simulink model "lqr_pos_control"  (R2021a)
settings: Solver=FixedStepAuto  StartTime=0.0  StopTime=inf  FixedStep=.01  RelTol=1e-3
model workspace (MAT data in the model file):
  SL_ROS_VariableLengthArrays_MaxSizes.CommonInfo.ArrayTruncateAction = 'EmitWarning'
  SL_ROS_VariableLengthArrays_MaxSizes.MsgTypeMap = containers.Map
  SL_ROS_VariableLengthArrays_MaxSizes.MsgTypeMap.serialization.keys = {'mav_msgs/Actuators'}
  SL_ROS_VariableLengthArrays_MaxSizes.MsgTypeMap.serialization.values{1}(1).PropertyName = 'Angles'
  SL_ROS_VariableLengthArrays_MaxSizes.MsgTypeMap.serialization.values{1}(1).DataType = 'double'
  SL_ROS_VariableLengthArrays_MaxSizes.MsgTypeMap.serialization.values{1}(1).MaxLength = 128
  SL_ROS_VariableLengthArrays_MaxSizes.MsgTypeMap.serialization.values{1}(2).PropertyName = 'AngularVelocities'
  SL_ROS_VariableLengthArrays_MaxSizes.MsgTypeMap.serialization.values{1}(2).DataType = 'double'
  SL_ROS_VariableLengthArrays_MaxSizes.MsgTypeMap.serialization.values{1}(2).MaxLength = 4
  SL_ROS_VariableLengthArrays_MaxSizes.MsgTypeMap.serialization.values{1}(3).PropertyName = 'Normalized'
  SL_ROS_VariableLengthArrays_MaxSizes.MsgTypeMap.serialization.values{1}(3).DataType = 'double'
  SL_ROS_VariableLengthArrays_MaxSizes.MsgTypeMap.serialization.values{1}(3).MaxLength = 128
  SL_ROS_VariableLengthArrays_MaxSizes.MsgTypeMap.serialization.uniformity = 0
  SL_ROS_VariableLengthArrays_MaxSizes.MsgTypeMap.serialization.keyType = 'char'
  SL_ROS_VariableLengthArrays_MaxSizes.MsgTypeMap.serialization.valueType = 'any'
values from neighbouring files (symbols this model uses):
  airframe = struct()    [discreteModel_initializer.m]
  Fs = 100    [discreteModel_initializer.m]
  g = 9.81    [discreteModel_initializer.m]
  kLQR = dlqr(lqrDiscrete.A,lqrDiscrete.B,Q,R)    [discreteModel_initializer.m]
  Ts = 1/Fs    (= 0.01)    [discreteModel_initializer.m]
  wiHover = sqrt(((airframe.mass)*9.81)/(4*airframe.Propeller.Ct))    [discreteModel_initializer.m]
undefined symbols (not defined in the file or in its folder): DiscIntNeverNeededParam, Discrete, Gyro_pitch, Gyro_roll, P00, P01, P11, Qkalman, Rkalman, RPM_to_DC, rpmKnown_throttleUnknown, sigbuilder_block, tf1, Time
libraries: robotlib x11, arduinolib x6, sharedtransform x3, simulink x3, ctrlSharedLib x1
(part 1 of 2)
settings Model: SILPILModeSetting=veronly  EnablePacing=on  ExtModeTrigDuration=2  Creator=aaron  LastModifiedBy=aaron
settings OptimizationCC: EnhancedBackFolding=on  PassReuseOutputArgsAs=Individual arguments  ZeroExternalMemoryAtStartup=off  ZeroInternalMemoryAtStartup=off  MaxStackSize=64  OptimizeBlockOrder=speed  DifferentSizesBufferReuse=on  OptimizationCustomize=off  EfficientTunableParamExpr=on
settings DebuggingCC: ParameterTunabilityLossMsg=error  UnderSpecifiedDimensionMsg=warning
settings HardwareCC: ProdBitPerPointer=32  ProdBitPerSizeT=32  ProdBitPerPtrDiffT=32  ProdLargestAtomicFloat=None  ProdIntDivRoundTo=Undefined  ProdEndianess=Unspecified  ProdWordSize=32  ProdHWDeviceType=Generic->Unspecified (assume 32-bit Generic)
settings SFSimCC: MATLABDynamicMemAlloc=off
settings RTWCC: SystemTargetFile=ert.tlc  HardwareBoard=Robot Operating System (ROS)  TLCOptions="-aInlineSetEventsForThisBaseRateFcn=TLC_FALSE -aSuppressMultiTaskScheduler=TLC_FALSE    -aRateBasedStepFcn=0"  TemplateMakefile=ert_default_tmf  Toolchain=Catkin  BuildConfiguration=Faster Runs  TargetLang=C++
settings CodeAppCC: ForceParamTrailComments=on  IgnoreCustomStorageClasses=off  OperatorAnnotations=on  SimulinkDataObjDesc=on  SFDataObjDesc=on  InsertBlockDesc=on
settings ERTTargetCC: SupportContinuousTime=on  ExtModeStaticAllocSize=24576

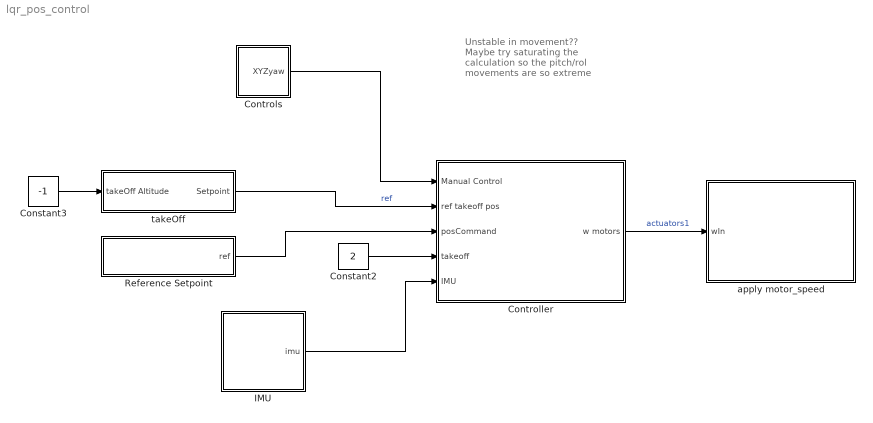
== system lqr_pos_control ==
  note: Unstable in movement??
      | Maybe try saturating the calculation so the pitch/rol movements are so extreme
  Constant2 : Constant  Value=2
  Constant3 : Constant  Value=-1
  Controller : Subsystem
  Controls : Subsystem
  IMU : Subsystem
  Reference Setpoint : Subsystem
  apply motor_speed : Subsystem
  takeOff : Subsystem
  wires:
  Controls/1(XYZyaw) -> Controller/1(Manual Control)
  takeOff/1(Setpoint) -> Controller/2(ref takeoff pos)  "ref"
  Constant3/1 -> takeOff/1(takeOff Altitude)
  Controller/1(w motors) -> apply motor_speed/1(wIn)  "actuators1"
  Constant2/1 -> Controller/4(takeoff)
  IMU/1(imu) -> Controller/5(IMU)
  Reference Setpoint/1(ref) -> Controller/3(posCommand)

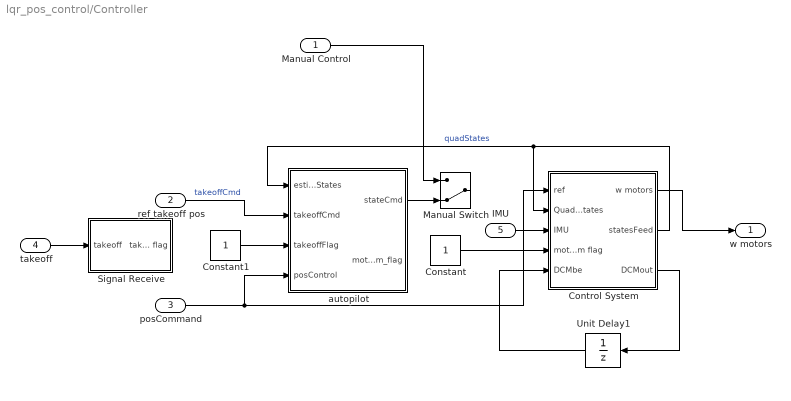
== system lqr_pos_control/Controller ==
  Manual Control : Inport
  ref takeoff pos : Inport  Port=2
  posCommand : Inport  Port=3
  takeoff : Inport  Port=4
  IMU : Inport  Port=5
  Constant : Constant
  Constant1 : Constant
  Control System : Subsystem
  Manual Switch : ManualSwitch  CurrentSetting=0
  Signal Receive : Subsystem
  Unit Delay1 : UnitDelay  InitialCondition=eye(3)  SampleTime=-1  HasFrameUpgradeWarning=on
  autopilot : Stateflow chart  TreatAsAtomicUnit=on
  w motors : Outport
  wires:
  autopilot/1(stateCmd) -> Manual Switch/2
  Manual Control/1 -> Manual Switch/1
  Control System/3(DCMout) -> Unit Delay1/1
  Control System/1(w motors) -> w motors/1
  IMU/1 -> Control System/3(IMU)
  posCommand/1 -> Control System/1(ref), autopilot/4(posControl)
  ref takeoff pos/1 -> autopilot/2(takeoffCmd)  "takeoffCmd"
  Control System/2(statesFeed) -> Control System/2(Quad States), autopilot/1(estimatedStates)  "quadStates"
  Unit Delay1/1 -> Control System/5(DCMbe)
  takeoff/1 -> Signal Receive/1(takeoff)
  Constant/1 -> Control System/4(motor arm flag)
  Constant1/1 -> autopilot/3(takeoffFlag)

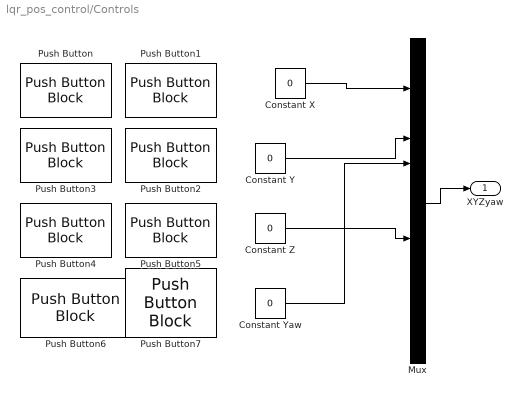
== system lqr_pos_control/Controls ==
  Constant X : Constant  Value=0
  Constant Y : Constant  Value=0
  Constant Yaw : Constant  Value=0
  Constant Z : Constant  Value=0
  Mux : Mux  Inputs=12
  Push Button : PushButtonBlock  LabelPosition=Top  ButtonText=Forward
  Push Button1 : PushButtonBlock  LabelPosition=Top  ButtonText=Backward  OnValue=-1
  Push Button2 : PushButtonBlock  LabelPosition=Top  ButtonText=Right
  Push Button3 : PushButtonBlock  LabelPosition=Top  ButtonText=Left  OnValue=-1
  Push Button4 : PushButtonBlock  LabelPosition=Top  ButtonText=Down  OnValue=-3
  Push Button5 : PushButtonBlock  LabelPosition=Top  ButtonText=Up  OnValue=3
  Push Button6 : PushButtonBlock  LabelPosition=Top  ButtonText=Counterclockwise  OnValue=-1
  Push Button7 : PushButtonBlock  LabelPosition=Top  ButtonText=Clockwise
  XYZyaw : Outport
  wires:
  Mux/1 -> XYZyaw/1
  Constant Yaw/1 -> Mux/5
  Constant X/1 -> Mux/2
  Constant Y/1 -> Mux/4
  Constant Z/1 -> Mux/8

== system lqr_pos_control/IMU ==
  Gain : Gain  Gain=-1
  Mux : Mux  Inputs=6
  Subscribe : robotlib/Subscribe  topicSource=Select from ROS network  topic=/hummingbird/imu  messageType=sensor_msgs/Imu  SampleTime=-1  legacyBusStruct=off  messageQueueLength=1
  Subsystem : Subsystem
  imu : Outport
  wires:
  Subsystem/5(<Y>1) -> Mux/5
  Subsystem/2(<Y>) -> Mux/2
  Subsystem/4(<X>1) -> Mux/4
  Subsystem/6(<Z>1) -> Mux/6
  Subscribe/1 -> Subsystem/Enable
  Subsystem/3(<Z>) -> Gain/1
  Subsystem/1(<X>) -> Mux/1
  Gain/1 -> Mux/3
  Subscribe/2 -> Subsystem/1(In1)
  Mux/1 -> imu/1  "imu"

== system lqr_pos_control/Reference Setpoint ==
  Subscribe4 : robotlib/Subscribe  topicSource=Select from ROS network  topic=/hummingbird/command/pose  messageType=geometry_msgs/PoseStamped  SampleTime=-1  legacyBusStruct=off  messageQueueLength=1
  Subsystem4 : Subsystem
  posControl : Subsystem
  ref : Outport
  wires:
  Subsystem4/3(cmdZ) -> posControl/3(cmdZ)
  Subsystem4/1(cmdX) -> posControl/1(cmdX)
  Subsystem4/4(quatOut) -> posControl/4(cmdAngle)
  Subscribe4/2 -> Subsystem4/1(In1)
  Subscribe4/1 -> Subsystem4/Enable
  Subsystem4/2(cmdY) -> posControl/2(cmdY)
  posControl/1(Setpoint) -> ref/1  "ref"

== system lqr_pos_control/apply motor_speed ==
  wIn : Inport
  MATLAB Function : MATLAB Function  TreatAsAtomicUnit=on
  Publish1 : robotlib/Publish  topicSource=Select from ROS network  topic=/hummingbird/command/motor_speed  messageType=mav_msgs/Actuators  legacyBusStruct=off  messageQueueLength=1
  Subscribe : robotlib/Subscribe  topicSource=Select from ROS network  topic=/hummingbird/motor_speed  messageType=mav_msgs/Actuators  SampleTime=-1  legacyBusStruct=off  messageQueueLength=1
  Subsystem : Subsystem
  wires:
  Subscribe/2 -> Subsystem/1(In1)
  Subscribe/1 -> Subsystem/Enable
  wIn/1 -> MATLAB Function/2(angVel)
  Subsystem/1(<AngularVelocities>) -> MATLAB Function/1(Bus)
  MATLAB Function/1(msg) -> Publish1/1

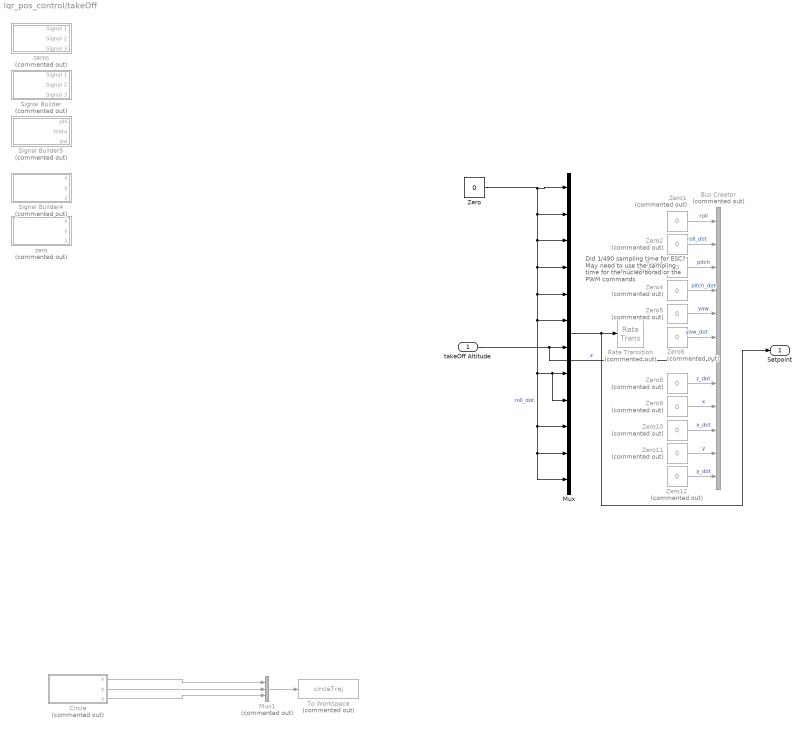
== system lqr_pos_control/takeOff ==
  note: Did 1/490 sampling time for ESC? May need to use the sampling time
      | for the nucleo borad or the PWM commands
  takeOff Altitude : Inport
  Bus Creator : BusCreator  Commented=on  Inputs=12
  Circle : Subsystem  Tag=STV Subsys  Commented=on  LoadFcn=sigbuilder_block('load');  StartFcn=sigbuilder_block('start');  StopFcn=sigbuilder_block('stop');  ClipboardFcn=sigbuilder_block('clipboard');  mask(Sigbuilder block){tuvar=[0:10]}
      mask help: Simulink:masks:SigbuilderBlock_MD
      mask init:
      | if ~strcmp(get_param(bdroot(gcbh),'SimulationStatus'),'stopped') tuvar = sigbuilder_block('maskInit'); end
      settings: CopyFcn=sigbuilder_block('copy');  DeleteFcn=sigbuilder_block('delete');  ModelCloseFcn=sigbuilder_block('modelClose');  PreSaveFcn=sigbuilder_block('preSave');  PauseFcn=sigbuilder_block('pause');  ContinueFcn=sigbuilder_block('continue');  NameChangeFcn=sigbuilder_block('namechange');  OpenFcn=sigbuilder_block('open',[792 346.5 550.5 399.75 ]);  CloseFcn=sigbuilder_block('close');
      mask Display: plot(0, 0, 100, 100,[2, 2, 32, 32, 2], [68, 8, 8, 68, 68],[32, 2], [38, 38], [32, 19, 2],[53, 60, 44], [32, 17, 17, 2],[16, 16, 31, 31]);txt = getActiveGroup(gcbh);text(2, 100, txt,'verticalAlignment', 'top');
  Mux : Mux  Inputs=12
  Mux1 : Mux  Commented=on  Inputs=3
  Rate Transition : RateTransition  Commented=on  OutPortSampleTime=1/490
  Signal Builder : Subsystem  Tag=STV Subsys  Commented=on  LoadFcn=sigbuilder_block('load');  StartFcn=sigbuilder_block('start');  StopFcn=sigbuilder_block('stop');  ClipboardFcn=sigbuilder_block('clipboard');  mask(Sigbuilder block){tuvar=[0:10]}
      mask help: Simulink:masks:SigbuilderBlock_MD
      mask init:
      | if ~strcmp(get_param(bdroot(gcbh),'SimulationStatus'),'stopped') tuvar = sigbuilder_block('maskInit'); end
      settings: CopyFcn=sigbuilder_block('copy');  DeleteFcn=sigbuilder_block('delete');  ModelCloseFcn=sigbuilder_block('modelClose');  PreSaveFcn=sigbuilder_block('preSave');  PauseFcn=sigbuilder_block('pause');  ContinueFcn=sigbuilder_block('continue');  NameChangeFcn=sigbuilder_block('namechange');  OpenFcn=sigbuilder_block('open',[437.6 199.2 550.4 400 ]);  CloseFcn=sigbuilder_block('close');
      mask Display: plot(0, 0, 100, 100,[2, 2, 32, 32, 2], [68, 8, 8, 68, 68],[32, 2], [38, 38], [32, 19, 2],[53, 60, 44], [32, 17, 17, 2],[16, 16, 31, 31]);txt = getActiveGroup(gcbh);text(2, 100, txt,'verticalAlignment', 'top');
  Signal Builder4 : Subsystem  Tag=STV Subsys  Commented=on  LoadFcn=sigbuilder_block('load');  StartFcn=sigbuilder_block('start');  StopFcn=sigbuilder_block('stop');  ClipboardFcn=sigbuilder_block('clipboard');  mask(Sigbuilder block){tuvar=[0:10]}
      mask help: Simulink:masks:SigbuilderBlock_MD
      mask init:
      | if ~strcmp(get_param(bdroot(gcbh),'SimulationStatus'),'stopped') tuvar = sigbuilder_block('maskInit'); end
      settings: CopyFcn=sigbuilder_block('copy');  DeleteFcn=sigbuilder_block('delete');  ModelCloseFcn=sigbuilder_block('modelClose');  PreSaveFcn=sigbuilder_block('preSave');  PauseFcn=sigbuilder_block('pause');  ContinueFcn=sigbuilder_block('continue');  NameChangeFcn=sigbuilder_block('namechange');  OpenFcn=sigbuilder_block('open',[437.6 199.2 550.4 400 ]);  CloseFcn=sigbuilder_block('close');
      mask Display: plot(0, 0, 100, 100,[2, 2, 32, 32, 2], [68, 8, 8, 68, 68],[32, 2], [38, 38], [32, 19, 2],[53, 60, 44], [32, 17, 17, 2],[16, 16, 31, 31]);txt = getActiveGroup(gcbh);text(2, 100, txt,'verticalAlignment', 'top');
  Signal Builder5 : Subsystem  Tag=STV Subsys  Commented=on  LoadFcn=sigbuilder_block('load');  StartFcn=sigbuilder_block('start');  StopFcn=sigbuilder_block('stop');  ClipboardFcn=sigbuilder_block('clipboard');  mask(Sigbuilder block){tuvar=[0:10]}
      mask help: Simulink:masks:SigbuilderBlock_MD
      mask init:
      | if ~strcmp(get_param(bdroot(gcbh),'SimulationStatus'),'stopped') tuvar = sigbuilder_block('maskInit'); end
      settings: CopyFcn=sigbuilder_block('copy');  DeleteFcn=sigbuilder_block('delete');  ModelCloseFcn=sigbuilder_block('modelClose');  PreSaveFcn=sigbuilder_block('preSave');  PauseFcn=sigbuilder_block('pause');  ContinueFcn=sigbuilder_block('continue');  NameChangeFcn=sigbuilder_block('namechange');  OpenFcn=sigbuilder_block('open',[6 30.75 1428 681.75 ]);  CloseFcn=sigbuilder_block('close');
      mask Display: plot(0, 0, 100, 100,[2, 2, 32, 32, 2], [68, 8, 8, 68, 68],[32, 2], [38, 38], [32, 19, 2],[53, 60, 44], [32, 17, 17, 2],[16, 16, 31, 31]);txt = getActiveGroup(gcbh);text(2, 100, txt,'verticalAlignment', 'top');
  To Workspace : ToWorkspace  Commented=on  VariableName=circleTraj  SampleTime=-1
  Zero : Constant  Value=0  OutDataTypeStr=Inherit: Inherit via back propagation
  Zero{1..6,8..12} (11 alike) : Constant  Commented=on  Value=0  OutDataTypeStr=Inherit: Inherit via back propagation
  zero : Subsystem  Tag=STV Subsys  Commented=on  LoadFcn=sigbuilder_block('load');  StartFcn=sigbuilder_block('start');  StopFcn=sigbuilder_block('stop');  ClipboardFcn=sigbuilder_block('clipboard');  mask(Sigbuilder block){tuvar=[0:10]}
      mask help: Simulink:masks:SigbuilderBlock_MD
      mask init:
      | if ~strcmp(get_param(bdroot(gcbh),'SimulationStatus'),'stopped') tuvar = sigbuilder_block('maskInit'); end
      settings: CopyFcn=sigbuilder_block('copy');  DeleteFcn=sigbuilder_block('delete');  ModelCloseFcn=sigbuilder_block('modelClose');  PreSaveFcn=sigbuilder_block('preSave');  PauseFcn=sigbuilder_block('pause');  ContinueFcn=sigbuilder_block('continue');  NameChangeFcn=sigbuilder_block('namechange');  OpenFcn=sigbuilder_block('open',[437.6 199.2 550.4 400 ]);  CloseFcn=sigbuilder_block('close');
      mask Display: plot(0, 0, 100, 100,[2, 2, 32, 32, 2], [68, 8, 8, 68, 68],[32, 2], [38, 38], [32, 19, 2],[53, 60, 44], [32, 17, 17, 2],[16, 16, 31, 31]);txt = getActiveGroup(gcbh);text(2, 100, txt,'verticalAlignment', 'top');
  zeros : Subsystem  Tag=STV Subsys  Commented=on  LoadFcn=sigbuilder_block('load');  StartFcn=sigbuilder_block('start');  StopFcn=sigbuilder_block('stop');  ClipboardFcn=sigbuilder_block('clipboard');  mask(Sigbuilder block){tuvar=[0:10]}
      mask help: Simulink:masks:SigbuilderBlock_MD
      mask init:
      | if ~strcmp(get_param(bdroot(gcbh),'SimulationStatus'),'stopped') tuvar = sigbuilder_block('maskInit'); end
      settings: CopyFcn=sigbuilder_block('copy');  DeleteFcn=sigbuilder_block('delete');  ModelCloseFcn=sigbuilder_block('modelClose');  PreSaveFcn=sigbuilder_block('preSave');  PauseFcn=sigbuilder_block('pause');  ContinueFcn=sigbuilder_block('continue');  NameChangeFcn=sigbuilder_block('namechange');  OpenFcn=sigbuilder_block('open',[6 30 1428 681.75 ]);  CloseFcn=sigbuilder_block('close');
      mask Display: plot(0, 0, 100, 100,[2, 2, 32, 32, 2], [68, 8, 8, 68, 68],[32, 2], [38, 38], [32, 19, 2],[53, 60, 44], [32, 17, 17, 2],[16, 16, 31, 31]);txt = getActiveGroup(gcbh);text(2, 100, txt,'verticalAlignment', 'top');
  Setpoint : Outport
  wires:
  Zero12/1 -> Bus Creator/12  "y_dot"
  Zero11/1 -> Bus Creator/11  "y"
  Zero10/1 -> Bus Creator/10  "x_dot"
  Zero9/1 -> Bus Creator/9  "x"
  Zero8/1 -> Bus Creator/8  "z_dot"
  Zero6/1 -> Bus Creator/6  "yaw_dot"
  Zero5/1 -> Bus Creator/5  "yaw"
  Zero4/1 -> Bus Creator/4  "pitch_dot"
  Zero3/1 -> Bus Creator/3  "pitch"
  Zero2/1 -> Bus Creator/2  "roll_dot"
  Zero1/1 -> Bus Creator/1  "roll"
  takeOff Altitude/1 -> Mux/7, Bus Creator/7  "z"
  Zero/1 -> Mux/1, Mux/2, Mux/3, Mux/4, Mux/6, Mux/9, Mux/8, Mux/11, Mux/12, Mux/10, Mux/5  "roll_dot"
  Mux/1 -> Setpoint/1, Rate Transition/1
  Circle/1(x) -> Mux1/1
  Circle/2(y) -> Mux1/2
  Mux1/1 -> To Workspace/1
  Circle/3(z) -> Mux1/3

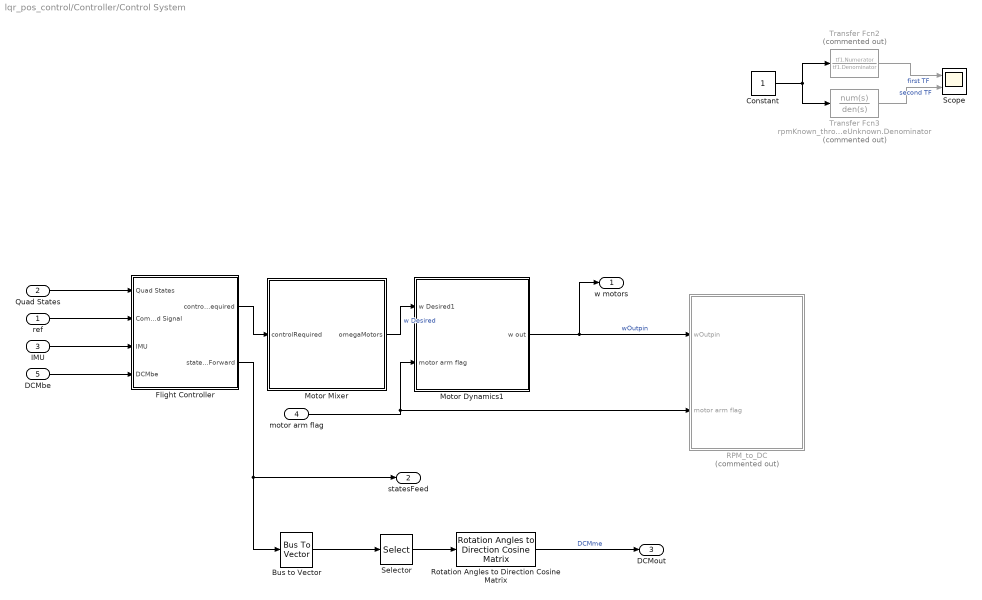
== system lqr_pos_control/Controller/Control System ==
  ref : Inport
  Quad States : Inport  Port=2
  IMU : Inport  Port=3
  motor arm flag : Inport  Port=4
  DCMbe : Inport  Port=5
  Bus to Vector : BusToVector
  Constant : Constant
  Flight Controller : Subsystem
  Motor Dynamics1 : Subsystem
  Motor Mixer : Subsystem
  RPM_to_DC : Subsystem  Commented=on
  Rotation Angles to Direction Cosine Matrix : sharedtransform/Rotation Angles to Direction Cosine Matrix  rotationOrder=ZYX  aMode=aMode
      settings: SourceProductBaseCode=AE,PW,DR,MT,UV,VE
  Scope : Scope  NumInputPorts=2
  Selector : Selector  InputPortWidth=12  IndexOptions=Index vector (dialog)  Indices=[5 3 1]  OutputSizes=1
  Transfer Fcn2 : TransferFcn  Commented=on  Numerator=tf1.Numerator  Denominator=tf1.Denominator
  Transfer Fcn3 : TransferFcn  Commented=on  Numerator=rpmKnown_throttleUnknown.Numerator  Denominator=rpmKnown_throttleUnknown.Denominator
  w motors : Outport
  statesFeed : Outport  Port=2
  DCMout : Outport  Port=3
  wires:
  Flight Controller/1(controlRequired) -> Motor Mixer/1(controlRequired)
  Quad States/1 -> Flight Controller/1(Quad States)
  IMU/1 -> Flight Controller/3(IMU)
  ref/1 -> Flight Controller/2(Command Signal)
  Motor Dynamics1/1(w out) -> RPM_to_DC/1(wOutpin), w motors/1  "wOutpin"
  Motor Mixer/1(omegaMotors) -> Motor Dynamics1/1(w Desired1)  "w Desired"
  motor arm flag/1 -> Motor Dynamics1/2(motor arm flag), RPM_to_DC/2(motor arm flag)
  DCMbe/1 -> Flight Controller/4(DCMbe)
  Constant/1 -> Transfer Fcn3/1, Transfer Fcn2/1
  Transfer Fcn2/1 -> Scope/1  "first TF"
  Transfer Fcn3/1 -> Scope/2  "second TF"
  Flight Controller/2(statesFeedForward) -> Bus to Vector/1, statesFeed/1
  Selector/1 -> Rotation Angles to Direction Cosine Matrix/1
  Rotation Angles to Direction Cosine Matrix/1 -> DCMout/1  "DCMme"
  Bus to Vector/1 -> Selector/1

== system lqr_pos_control/Controller/Signal Receive ==
  takeoff : Inport
  Compare To Constant : simulink/Logic and Bit Operations/Compare To Constant  relop===  const=2  OutDataTypeStr=boolean
  Compare To Constant3 : simulink/Logic and Bit Operations/Compare To Constant  relop===  const=1  OutDataTypeStr=boolean
  Constant : Constant
  Constant1 : Constant  Value=0
  Digital Output : arduinolib/Digital Output  Commented=on  pinNumber=13  Direction=output  blockPlatform=arduino
  Merge : Merge
  Rate Transition : RateTransition
  Serial Receive1 : arduinolib/Serial Receive  Commented=on  isARMArch=off  portNumber=1  DataType=uint8  Datalength=1  SampleTime=Ts  showOutStatus=on  blockPlatform=arduino
      settings: SourceProductBaseCode=ARDUINO
  Terminator : Terminator
  Triggered Subsystem : Subsystem  TreatAsAtomicUnit=on
  Triggered Subsystem1 : Subsystem  TreatAsAtomicUnit=on
  takeoff flag : Outport
  wires:
  Triggered Subsystem1/1(Out1) -> Merge/2
  Triggered Subsystem/1(Out1) -> Merge/1
  Constant1/1 -> Triggered Subsystem1/1(In1)
  Constant/1 -> Triggered Subsystem/1(In1)
  Compare To Constant/1 -> Triggered Subsystem/Trigger
  takeoff/1 -> Compare To Constant/1, Compare To Constant3/1
  Compare To Constant3/1 -> Triggered Subsystem1/Trigger
  Merge/1 -> Rate Transition/1, Digital Output/1  "COM7 COmmands"
  Serial Receive1/2 -> Terminator/1
  Rate Transition/1 -> takeoff flag/1

== system lqr_pos_control/IMU/Subsystem ==
  In1 : Inport
  Enable : EnablePort
  Blank Message : robotlib/Blank Message  Commented=on  messageClass=Service Request  entityType=std_srvs/Empty  messageType=std_srvs/EmptyRequest  SampleTime=inf  legacyBusStruct=off
  Bus Selector : BusSelector  OutputSignals=LinearAcceleration.X,LinearAcceleration.Y,LinearAcceleration.Z,AngularVelocity.X,AngularVelocity.Y,AngularVelocity.Z
  Call Service : robotlib/Call Service  Commented=on  topicSource=Select from ROS network  service=/gazebo/pause_physics  serviceType=std_srvs/Empty  connectionTimeout=5  keepPersistent=on  ShowErrorCodeOutput=on  legacyBusStruct=off
      settings: SourceProductBaseCode=RR
  <X> : Outport
  <Y> : Outport  Port=2
  <Z> : Outport  Port=3
  <X>1 : Outport  Port=4
  <Y>1 : Outport  Port=5
  <Z>1 : Outport  Port=6
  wires:
  Bus Selector/6 -> <Z>1/1  "<Z>"
  Bus Selector/5 -> <Y>1/1  "<Y>"
  Bus Selector/1 -> <X>/1  "<X>"
  Bus Selector/3 -> <Z>/1  "<Z>"
  Bus Selector/4 -> <X>1/1  "<X>"
  Bus Selector/2 -> <Y>/1  "<Y>"
  In1/1 -> Bus Selector/1
  Blank Message/1 -> Call Service/1

== system lqr_pos_control/Reference Setpoint/Subsystem4 ==
  In1 : Inport
  Enable : EnablePort
  Bus Selector : BusSelector  OutputSignals=Pose.Position.X,Pose.Position.Y,Pose.Position.Z,Pose.Orientation.X,Pose.Orientation.Y,Pose.Orientation.Z,Pose.Orientation.W
  Mux : Mux
  cmdX : Outport
  cmdY : Outport  Port=2
  cmdZ : Outport  Port=3
  quatOut : Outport  Port=4
  wires:
  Bus Selector/1 -> cmdX/1  "<X>"
  Bus Selector/2 -> cmdY/1  "<Y>"
  Bus Selector/3 -> cmdZ/1  "<Z>"
  In1/1 -> Bus Selector/1
  Bus Selector/4 -> Mux/2  "<X>"
  Bus Selector/7 -> Mux/1  "<W>"
  Bus Selector/5 -> Mux/3  "<Y>"
  Bus Selector/6 -> Mux/4  "<Z>"
  Mux/1 -> quatOut/1

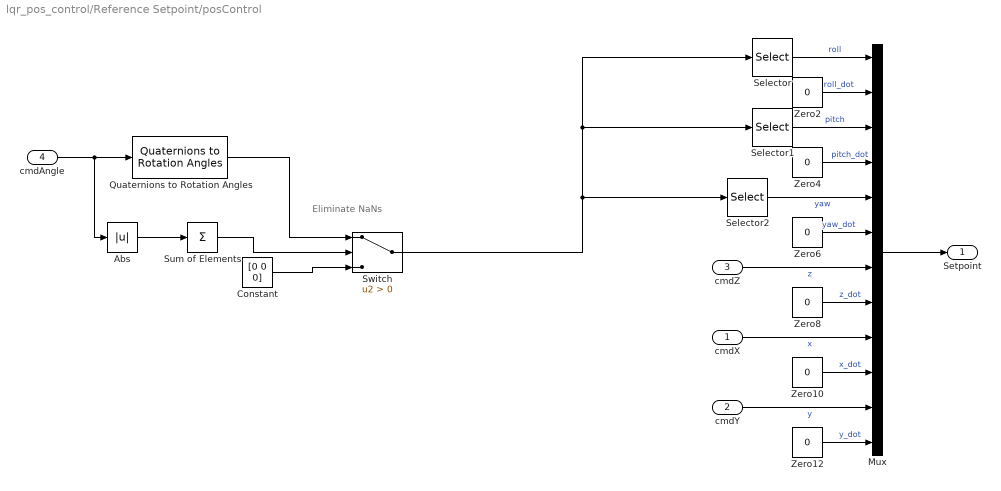
== system lqr_pos_control/Reference Setpoint/posControl ==
  note: Eliminate NaNs
  cmdX : Inport
  cmdY : Inport  Port=2
  cmdZ : Inport  Port=3
  cmdAngle : Inport  Port=4
  Abs : Abs
  Constant : Constant  Value=[0 0 0]
  Mux : Mux  Inputs=12
  Quaternions to Rotation Angles : sharedtransform/Quaternions to Rotation Angles  rotationOrder=ZYX  aMode=aMode
      settings: SourceProductBaseCode=AE,PW,DR,MT,UV,VE
  Selector : Selector  InputPortWidth=3  IndexOptions=Index vector (dialog)  Indices=1  OutputSizes=1
  Selector1 : Selector  InputPortWidth=3  IndexOptions=Index vector (dialog)  Indices=2  OutputSizes=1
  Selector2 : Selector  InputPortWidth=3  IndexOptions=Index vector (dialog)  Indices=3  OutputSizes=1
  Sum of Elements : Sum  Inputs=+
  Switch : Switch  Criteria=u2 > Threshold
  Zero{2,4,6,8,10,12} (6 alike) : Constant  Value=0  OutDataTypeStr=Inherit: Inherit via back propagation
  Setpoint : Outport
  wires:
  Selector/1 -> Mux/1  "roll"
  Zero2/1 -> Mux/2  "roll_dot"
  Selector1/1 -> Mux/3  "pitch"
  Zero4/1 -> Mux/4  "pitch_dot"
  Selector2/1 -> Mux/5  "yaw"
  Zero6/1 -> Mux/6  "yaw_dot"
  Zero8/1 -> Mux/8  "z_dot"
  cmdX/1 -> Mux/9  "x"
  Zero10/1 -> Mux/10  "x_dot"
  cmdY/1 -> Mux/11  "y"
  Zero12/1 -> Mux/12  "y_dot"
  cmdZ/1 -> Mux/7  "z"
  Mux/1 -> Setpoint/1
  cmdAngle/1 -> Abs/1, Quaternions to Rotation Angles/1
  Constant/1 -> Switch/3
  Quaternions to Rotation Angles/1 -> Switch/1
  Sum of Elements/1 -> Switch/2
  Abs/1 -> Sum of Elements/1
  Switch/1 -> Selector1/1, Selector/1, Selector2/1

== system lqr_pos_control/apply motor_speed/Subsystem ==
  In1 : Inport
  Enable : EnablePort
  Blank Message : robotlib/Blank Message  Commented=on  messageClass=Service Request  entityType=std_srvs/Empty  messageType=std_srvs/EmptyRequest  SampleTime=inf  legacyBusStruct=off
  Call Service : robotlib/Call Service  Commented=on  topicSource=Select from ROS network  service=/gazebo/unpause_physics  serviceType=std_srvs/Empty  connectionTimeout=5  keepPersistent=on  ShowErrorCodeOutput=on  legacyBusStruct=off
      settings: SourceProductBaseCode=RR
  <AngularVelocities> : Outport
  wires:
  In1/1 -> <AngularVelocities>/1
  Blank Message/1 -> Call Service/1

== system lqr_pos_control/takeOff/Circle ==
  Demux : Demux  Tag=STV Demux  Outputs=3
      settings: DisplayOption=none
  FromWs : FromWorkspace  Tag=STV FromWs  VariableName=tuvar
      SigBuilderData=|
      | common.afterFinalStr = 'Extrapolate'
      | common.sampleTime = 0
      | dataSet.timeRange = [0 60]
      | dataSet.name = 'Group 1'
      | sbobj.Groups.Name = 'Group 1'
      | sbobj.Groups.Signals(1).Name = 'x'
      | sbobj.Groups.Signals(1).XData = [0 0.005 0.01 0.015 0.02 0.025 0.03 0.035 0.04 0.045 0.05 0.055 ... (12001 elements, 1x12001)]
      | sbobj.Groups.Signals(1).YData = [0 0.0314158748588 0.0628314396556 0.0942463843314 0.125660398834 0.157073173118 0.188484397154 0.219893760925 0.251300954433 0.282705667703 0.314107590781 0.345506413745 ... (12001 elements, 1x12001)]
      | sbobj.Groups.Signals(2).Name = 'y'
      | sbobj.Groups.Signals(2).XData = [0 0.005 0.01 0.015 0.02 0.025 0.03 0.035 0.04 0.045 0.05 0.055 ... (12001 elements, 1x12001)]
      | sbobj.Groups.Signals(2).YData = [0 4.93479814185e-05 0.000197391438629 0.000444128910502 0.00078955796184 0.00123367518339 0.00177647619191 0.00241795563016 0.003158107167 0.00399692349743 0.00493439634268 0.00597051645027 ... (12001 elements, 1x12001)]
      | sbobj.Groups.Signals(3).Name = 'z'
      | sbobj.Groups.Signals(3).XData = [0 0.01 0.01 0.015 0.02 0.025 0.03 0.035 0.04 0.045 0.05 0.055 ... (12001 elements, 1x12001)]
      | sbobj.Groups.Signals(3).YData = [-0.25 -8.05 -7.99994078257 -7.99986676133 -7.99976313261 -7.99962989744 -7.99946705714 -7.99927461331 -7.99905256785 -7.99880092295 -7.9985196811 -7.99820884506 ... (12001 elements, 1x12001)]
      | sbobj.Groups.TimeRange = [0 60]
  x : Outport  Tag=STV Outport
  y : Outport  Tag=STV Outport  Port=2
  z : Outport  Tag=STV Outport  Port=3
  wires:
  FromWs/1 -> Demux/1
  Demux/1 -> x/1
  Demux/2 -> y/1
  Demux/3 -> z/1

== system lqr_pos_control/takeOff/Signal Builder ==
  Demux : Demux  Tag=STV Demux  Outputs=3
      settings: DisplayOption=none
  FromWs : FromWorkspace  Tag=STV FromWs  VariableName=tuvar
      SigBuilderData=|
      | common.afterFinalStr = 'Extrapolate'
      | common.sampleTime = 0
      | dataSet.timeRange = [0 60]
      | dataSet.name = 'Group 1'
      | sbobj.Groups.Name = 'Group 1'
      | sbobj.Groups.Signals(1).Name = 'Signal 1'
      | sbobj.Groups.Signals(1).XData = [0 4 4 30.1 30.1 60]
      | sbobj.Groups.Signals(1).YData = [0 0 1 1 0 0]
      | sbobj.Groups.Signals(2).Name = 'Signal 2'
      | sbobj.Groups.Signals(2).XData = [0 16.5 16.5 30.1 30.1 60]
      | sbobj.Groups.Signals(2).YData = [0 0 1 1 0 0]
      | sbobj.Groups.Signals(3).Name = 'Signal 3'
      | sbobj.Groups.Signals(3).XData = [0 24.6 24.6 40.9 40.9 60]
      | sbobj.Groups.Signals(3).YData = [0 0 1 1 0 0]
      | sbobj.Groups.TimeRange = [0 60]
  Signal 1 : Outport  Tag=STV Outport
  Signal 2 : Outport  Tag=STV Outport  Port=2
  Signal 3 : Outport  Tag=STV Outport  Port=3
  wires:
  Demux/1 -> Signal 1/1
  FromWs/1 -> Demux/1
  Demux/2 -> Signal 2/1
  Demux/3 -> Signal 3/1

== system lqr_pos_control/takeOff/Signal Builder4 ==
  Demux : Demux  Tag=STV Demux  Outputs=3
      settings: DisplayOption=none
  FromWs : FromWorkspace  Tag=STV FromWs  VariableName=tuvar
      SigBuilderData=|
      | common.afterFinalStr = 'Extrapolate'
      | common.sampleTime = 0
      | dataSet.timeRange = [0 30]
      | dataSet.name = 'Group 1'
      | sbobj.Groups.Name = 'Group 1'
      | sbobj.Groups.Signals(1).Name = 'x'
      | sbobj.Groups.Signals(1).XData = [0 3 15 30]
      | sbobj.Groups.Signals(1).YData = [0 0 100 0]
      | sbobj.Groups.Signals(2).Name = 'y'
      | sbobj.Groups.Signals(2).XData = [0 4 15 30]
      | sbobj.Groups.Signals(2).YData = [0 0 -100 0]
      | sbobj.Groups.Signals(3).Name = 'z'
      | sbobj.Groups.Signals(3).XData = [0 15 30]
      | sbobj.Groups.Signals(3).YData = [0 -50 0]
      | sbobj.Groups.TimeRange = [0 30]
  x : Outport  Tag=STV Outport
  y : Outport  Tag=STV Outport  Port=2
  z : Outport  Tag=STV Outport  Port=3
  wires:
  FromWs/1 -> Demux/1
  Demux/1 -> x/1
  Demux/2 -> y/1
  Demux/3 -> z/1

== system lqr_pos_control/takeOff/Signal Builder5 ==
  Demux : Demux  Tag=STV Demux  Outputs=3
      settings: DisplayOption=none
  FromWs : FromWorkspace  Tag=STV FromWs  VariableName=tuvar
      SigBuilderData=|
      | common.afterFinalStr = 'Extrapolate'
      | common.sampleTime = 0
      | dataSet.timeRange = [0 60]
      | dataSet.name = 'Group 1'
      | sbobj.Groups.Name = 'Group 1'
      | sbobj.Groups.Signals(1).Name = 'phi'
      | sbobj.Groups.Signals(1).XData = [0 3 10 10 20 20 50 50 60]
      | sbobj.Groups.Signals(1).YData = [0 0 0 0.2 0.2 0 0 0.2 0.2]
      | sbobj.Groups.Signals(2).Name = 'theta'
      | sbobj.Groups.Signals(2).XData = [0 10 20 30 30 40 40 60]
      | sbobj.Groups.Signals(2).YData = [0 0 0 0 0.2 0.2 0 0]
      | sbobj.Groups.Signals(3).Name = 'psi'
      | sbobj.Groups.Signals(3).XData = [0 5 5 10 10 20 60]
      | sbobj.Groups.Signals(3).YData = [0 0 0.5 0.5 0 0 0]
      | sbobj.Groups.TimeRange = [0 60]
  phi : Outport  Tag=STV Outport
  theta : Outport  Tag=STV Outport  Port=2
  psi : Outport  Tag=STV Outport  Port=3
  wires:
  FromWs/1 -> Demux/1
  Demux/1 -> phi/1
  Demux/2 -> theta/1
  Demux/3 -> psi/1

== system lqr_pos_control/takeOff/zero ==
  Demux : Demux  Tag=STV Demux  Outputs=3
      settings: DisplayOption=none
  FromWs : FromWorkspace  Tag=STV FromWs  VariableName=tuvar
      SigBuilderData=|
      | common.afterFinalStr = 'Extrapolate'
      | common.sampleTime = 0
      | dataSet.timeRange = [0 60]
      | dataSet.name = 'Group 1'
      | sbobj.Groups.Name = 'Group 1'
      | sbobj.Groups.Signals(1).Name = 'x'
      | sbobj.Groups.Signals(1).XData = [0 3 15 60]
      | sbobj.Groups.Signals(1).YData = [0 0 0 0]
      | sbobj.Groups.Signals(2).Name = 'y'
      | sbobj.Groups.Signals(2).XData = [0 4 15 60]
      | sbobj.Groups.Signals(2).YData = [0 0 0 0]
      | sbobj.Groups.Signals(3).Name = 'z'
      | sbobj.Groups.Signals(3).XData = [0 15 60]
      | sbobj.Groups.Signals(3).YData = [0 0 0]
      | sbobj.Groups.TimeRange = [0 60]
  x : Outport  Tag=STV Outport
  y : Outport  Tag=STV Outport  Port=2
  z : Outport  Tag=STV Outport  Port=3
  wires:
  FromWs/1 -> Demux/1
  Demux/1 -> x/1
  Demux/2 -> y/1
  Demux/3 -> z/1

== system lqr_pos_control/takeOff/zeros ==
  Demux : Demux  Tag=STV Demux  Outputs=3
      settings: DisplayOption=none
  FromWs : FromWorkspace  Tag=STV FromWs  VariableName=tuvar
      SigBuilderData=|
      | common.afterFinalStr = 'Extrapolate'
      | common.sampleTime = 0
      | dataSet.timeRange = [0 60]
      | dataSet.name = 'Group 1'
      | sbobj.Groups.Name = 'Group 1'
      | sbobj.Groups.Signals(1).Name = 'Signal 1'
      | sbobj.Groups.Signals(1).XData = [0 4 30.1 60]
      | sbobj.Groups.Signals(1).YData = [0 0 0 0]
      | sbobj.Groups.Signals(2).Name = 'Signal 2'
      | sbobj.Groups.Signals(2).XData = [0 16.5 30.1 60]
      | sbobj.Groups.Signals(2).YData = [0 0 0 0]
      | sbobj.Groups.Signals(3).Name = 'Signal 3'
      | sbobj.Groups.Signals(3).XData = [0 5 5.55 8.25 60]
      | sbobj.Groups.Signals(3).YData = [0 0 0 0 0]
      | sbobj.Groups.TimeRange = [0 60]
  Signal 1 : Outport  Tag=STV Outport
  Signal 2 : Outport  Tag=STV Outport  Port=2
  Signal 3 : Outport  Tag=STV Outport  Port=3
  wires:
  Demux/1 -> Signal 1/1
  FromWs/1 -> Demux/1
  Demux/2 -> Signal 2/1
  Demux/3 -> Signal 3/1

== system lqr_pos_control/Controller/Control System/Flight Controller ==
  Quad States : Inport
  Command Signal : Inport  Port=2
  IMU : Inport  Port=3
  DCMbe : Inport  Port=4
  Linear Controller : Subsystem
  State Estimation : Subsystem
  controlRequired : Outport
  statesFeedForward : Outport  Port=2
  wires:
  Command Signal/1 -> Linear Controller/1(Command Signal)
  State Estimation/1(State Estimation) -> statesFeedForward/1, Linear Controller/2(State Estimate)  "states"
  Linear Controller/1(controlRequired) -> controlRequired/1
  Quad States/1 -> State Estimation/1(Quad States)
  IMU/1 -> State Estimation/2(IMU)
  DCMbe/1 -> State Estimation/3(DCMbe)

== system lqr_pos_control/Controller/Control System/Motor Dynamics1 ==
  note: https://ctms.engin.umich.edu/CTMS/index.php?example=MotorSpeed&section=SimulinkModeling
  w Desired1 : Inport  SampleTime=Ts
  motor arm flag : Inport  Port=2
  Discrete-Time Integrator1 : DiscreteIntegrator  InitialCondition=wiHover*9.549297  SampleTime=Ts  ICPrevOutput=DiscIntNeverNeededParam  ICPrevScaledInput=DiscIntNeverNeededParam
  Gain1 : Gain  Gain=20
  Gain3 : Gain  Gain=1/9.549297
  Output Motor Speeds : Subsystem
  Quantizer4 : Quantizer  QuantizationInterval=5
  Saturation4 : Saturate  UpperLimit=8002  LowerLimit=0
  SignedSqrt1 : Sqrt  Operator=signedSqrt  IntermediateResultsDataTypeStr=single  SaturateOnIntegerOverflow=on
  Sum2 : Sum  Inputs=|+-
  convToRPM1 : Gain  Gain=9.549297
  w out : Outport  SampleTime=Ts
  wires:
  SignedSqrt1/1 -> convToRPM1/1  "wDesired"
  Discrete-Time Integrator1/1 -> Saturation4/1  "wactual"
  w Desired1/1 -> SignedSqrt1/1  "desired"
  Sum2/1 -> Gain1/1
  Saturation4/1 -> Gain3/1, Sum2/2
  Gain1/1 -> Discrete-Time Integrator1/1
  Gain3/1 -> Quantizer4/1  "ODE"
  convToRPM1/1 -> Sum2/1
  Quantizer4/1 -> Output Motor Speeds/2(ODE)  "ODE"
  motor arm flag/1 -> Output Motor Speeds/1(In1)
  Output Motor Speeds/1(Out1) -> w out/1

== system lqr_pos_control/Controller/Control System/Motor Mixer ==
  controlRequired : Inport
  Matrix Multiply : Product  Multiplication=Matrix(*)
  Rate Transition : RateTransition
  Variant Subsystem : Subsystem  Variant=on
  omegaMotors : Outport
  wires:
  Variant Subsystem/1(motorMixing) -> Matrix Multiply/1
  Matrix Multiply/1 -> Rate Transition/1  "thrustDesired"
  controlRequired/1 -> Matrix Multiply/2
  Rate Transition/1 -> omegaMotors/1

== system lqr_pos_control/Controller/Control System/RPM_to_DC ==
  wOutpin : Inport
  motor arm flag : Inport  Port=2
  Selector : Selector  InputPortWidth=4  IndexOptions=Index vector (dialog)  Indices=[1]  OutputSizes=1
  Selector1 : Selector  InputPortWidth=4  IndexOptions=Index vector (dialog)  Indices=[2]  OutputSizes=1
  Selector2 : Selector  InputPortWidth=4  IndexOptions=Index vector (dialog)  Indices=[3]  OutputSizes=1
  Selector3 : Selector  InputPortWidth=4  IndexOptions=Index vector (dialog)  Indices=[4]  OutputSizes=1
  Subsystem : Subsystem
  Subsystem1 : Subsystem
  Subsystem2 : Subsystem
  Subsystem3 : Subsystem
  convToRPM : Gain  Gain=9.549297
  wires:
  wOutpin/1 -> convToRPM/1
  convToRPM/1 -> Selector/1, Selector3/1, Selector2/1, Selector1/1
  Selector/1 -> Subsystem/1(In1)
  motor arm flag/1 -> Subsystem3/2(motor arm flag), Subsystem2/2(motor arm flag), Subsystem1/2(motor arm flag), Subsystem/2(motor arm flag)
  Selector1/1 -> Subsystem1/1(In1)
  Selector2/1 -> Subsystem2/1(In1)
  Selector3/1 -> Subsystem3/1(In1)

== system lqr_pos_control/Controller/Signal Receive/Triggered Subsystem ==
  In1 : Inport
  Trigger : TriggerPort  VariantControl=(inherit)
  Blank Message : robotlib/Blank Message  messageClass=Service Request  entityType=std_srvs/Empty  messageType=std_srvs/EmptyRequest  SampleTime=inf  legacyBusStruct=off
  Call Service : robotlib/Call Service  topicSource=Specify your own  service=/gazebo/unpause_physics  serviceType=std_srvs/Empty  connectionTimeout=5  keepPersistent=off  ShowErrorCodeOutput=on  legacyBusStruct=off
      settings: SourceProductBaseCode=RR
  Out1 : Outport
  wires:
  In1/1 -> Out1/1
  Blank Message/1 -> Call Service/1

== system lqr_pos_control/Controller/Signal Receive/Triggered Subsystem1 ==
  In1 : Inport
  Trigger : TriggerPort  VariantControl=(inherit)
  Out1 : Outport
  wires:
  In1/1 -> Out1/1

== system lqr_pos_control/Controller/Control System/Flight Controller/Linear Controller ==
  Command Signal : Inport
  State Estimate : Inport  Port=2
  Bus to Vector : BusToVector
  Constant : Constant  Value=g*(airframe.mass)  SampleTime=1/Fs
  Delay One Step : Delay  DelayLength=1
  Delay One Step1 : Delay  Commented=through  DelayLength=1  InitialCondition=[0 0 0 0]
  Demux : Demux
  Gain : Gain  Gain=-kLQR  Multiplication=Matrix(K*u)
  Mux : Mux
  Selector : Selector  InputPortWidth=4  IndexOptions=Index vector (dialog)  Indices=1  OutputSizes=1
  Sum : Sum  Inputs=|++
  Sum1 : Sum  Inputs=-+|
  controlRequired : Outport
  wires:
  Sum1/1 -> Gain/1
  State Estimate/1 -> Bus to Vector/1
  Delay One Step/1 -> Sum1/2
  Command Signal/1 -> Sum1/1
  Gain/1 -> Selector/1, Delay One Step1/1
  Selector/1 -> Sum/1  "Thrust needed"
  Delay One Step1/1 -> Demux/1
  Demux/4 -> Mux/4
  Mux/1 -> controlRequired/1  "controlNeeded"
  Sum/1 -> Mux/1  "totalThrustNeeded"
  Constant/1 -> Sum/2
  Demux/2 -> Mux/2
  Demux/3 -> Mux/3
  Bus to Vector/1 -> Delay One Step/1

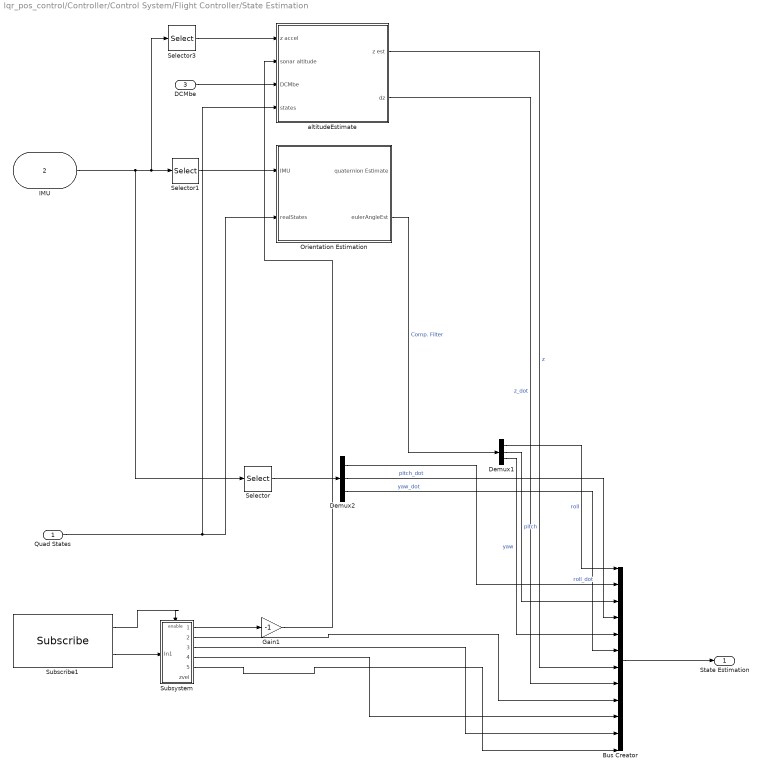
== system lqr_pos_control/Controller/Control System/Flight Controller/State Estimation ==
  Quad States : Inport
  IMU : Inport  Port=2
  DCMbe : Inport  Port=3
  Bus Creator : BusCreator  Inputs=12  OutDataTypeStr=Bus: stateCommand
  Demux1 : Demux  Outputs=3
  Demux2 : Demux  Outputs=3
  Gain1 : Gain  Gain=-1
  Orientation Estimation : Subsystem
  Selector : Selector  IndexOptions=Index vector (dialog)  Indices=[4 5 6]  OutputSizes=1
  Selector1 : Selector  InputPortWidth=6  IndexOptions=Index vector (dialog)  Indices=[1:6]  OutputSizes=1
  Selector3 : Selector  InputPortWidth=6  IndexOptions=Index vector (dialog)  Indices=[3]  OutputSizes=1
  Subscribe1 : robotlib/Subscribe  topicSource=Select from ROS network  topic=/hummingbird/ground_truth/odometry  messageType=nav_msgs/Odometry  SampleTime=-1  legacyBusStruct=off  messageQueueLength=1
  Subsystem : Subsystem
  altitudeEstimate : Subsystem
  State Estimation : Outport
  wires:
  Orientation Estimation/2(eulerAngleEst) -> Demux1/1  "Comp. Filter"
  Quad States/1 -> altitudeEstimate/4(states), Orientation Estimation/2(realStates)
  Selector/1 -> Demux2/1
  Demux2/1 -> Bus Creator/2  "roll_dot"
  Demux2/2 -> Bus Creator/4  "pitch_dot"
  Demux2/3 -> Bus Creator/6  "yaw_dot"
  Demux1/1 -> Bus Creator/1  "roll"
  Demux1/2 -> Bus Creator/3  "pitch"
  Demux1/3 -> Bus Creator/5  "yaw"
  IMU/1 -> Selector/1, Selector3/1, Selector1/1
  Selector1/1 -> Orientation Estimation/1(IMU)
  Selector3/1 -> altitudeEstimate/1(z accel)
  DCMbe/1 -> altitudeEstimate/3(DCMbe)
  altitudeEstimate/1(z est) -> Bus Creator/7  "z"
  altitudeEstimate/2(dz) -> Bus Creator/8  "z_dot"
  Bus Creator/1 -> State Estimation/1
  Subscribe1/2 -> Subsystem/1(In1)
  Subscribe1/1 -> Subsystem/Enable
  Subsystem/1(<Z>) -> Gain1/1
  Subsystem/5(<YVel>) -> Bus Creator/12
  Subsystem/4(<Xvel>1) -> Bus Creator/10
  Subsystem/3(<YPos>) -> Bus Creator/11
  Subsystem/2(<XPos>) -> Bus Creator/9
  Gain1/1 -> altitudeEstimate/2(sonar altitude)

== system lqr_pos_control/Controller/Control System/Motor Dynamics1/Output Motor Speeds ==
  In1 : Inport
  ODE : Inport  Port=2
  Demux : Demux
  Mux : Mux
  Step : Step  Time=.5  After=0  SampleTime=1/Fs
  Switch{,1..3} (4 alike) : Switch  Threshold=1
  Out1 : Outport
  wires:
  Switch3/1 -> Mux/4  "duty"
  In1/1 -> Switch3/2, Switch2/2, Switch1/2, Switch/2
  Step/1 -> Switch1/3, Switch3/3, Switch/3, Switch2/3
  Switch1/1 -> Mux/2  "duty"
  Demux/2 -> Switch1/1
  Demux/1 -> Switch/1
  Switch2/1 -> Mux/3  "duty"
  Demux/4 -> Switch3/1
  Demux/3 -> Switch2/1
  Switch/1 -> Mux/1  "duty"
  ODE/1 -> Demux/1
  Mux/1 -> Out1/1

== system lqr_pos_control/Controller/Control System/Motor Mixer/Variant Subsystem ==
  note: plusConfig == 1 FOR PLUS CONFIGURATION
      | plusConfig == 0 FOR X CONFIGURATION
  Plus Configuration : Subsystem  VariantControl=plusConfig == 1
  Plus Configuration2 : Subsystem  VariantControl=plusConfig == 2
  X Configuration : Subsystem  VariantControl=plusConfig == 0
  motorMixing : Outport

== system lqr_pos_control/Controller/Control System/RPM_to_DC/Subsystem ==
  In1 : Inport
  motor arm flag : Inport  Port=2
  Gain4 : Gain  Gain=2.55
  PWM4 : arduinolib/PWM  pinNumber=2  frequencyType=Specify  desiredFrequency=490.2  achievableFrequency=490.2
  Rate Transition : RateTransition
  Step : Step  Time=.5  Before=99  SampleTime=1/Fs
  Switch : Switch  Threshold=1
  Transfer Fcn1 : TransferFcn  Numerator=RPM_to_DC.Numerator  Denominator=RPM_to_DC.Denominator
  wires:
  Transfer Fcn1/1 -> Rate Transition/1  "testTF"
  Gain4/1 -> PWM4/1
  Step/1 -> Switch/3
  Rate Transition/1 -> Switch/1  "cont. duty"
  motor arm flag/1 -> Switch/2
  In1/1 -> Transfer Fcn1/1
  Switch/1 -> Gain4/1  "duty"

== system lqr_pos_control/Controller/Control System/RPM_to_DC/Subsystem1 ==
  In1 : Inport
  motor arm flag : Inport  Port=2
  Gain4 : Gain  Gain=2.55
  PWM4 : arduinolib/PWM  pinNumber=3  frequencyType=Specify  desiredFrequency=490.2  achievableFrequency=490.2
  Rate Transition : RateTransition
  Step : Step  Time=.5  Before=99  SampleTime=1/Fs
  Switch : Switch  Threshold=1
  Transfer Fcn1 : TransferFcn  Numerator=RPM_to_DC.Numerator  Denominator=RPM_to_DC.Denominator
  wires:
  Switch/1 -> Gain4/1  "duty"
  In1/1 -> Transfer Fcn1/1
  motor arm flag/1 -> Switch/2
  Rate Transition/1 -> Switch/1  "cont. duty"
  Step/1 -> Switch/3
  Gain4/1 -> PWM4/1
  Transfer Fcn1/1 -> Rate Transition/1  "testTF"

== system lqr_pos_control/Controller/Control System/RPM_to_DC/Subsystem2 ==
  In1 : Inport
  motor arm flag : Inport  Port=2
  Gain4 : Gain  Gain=2.55
  PWM4 : arduinolib/PWM  pinNumber=4  frequencyType=Specify  desiredFrequency=490.2  achievableFrequency=490.2
  Rate Transition : RateTransition
  Step : Step  Time=.5  Before=99  SampleTime=1/Fs
  Switch : Switch  Threshold=1
  Transfer Fcn1 : TransferFcn  Numerator=RPM_to_DC.Numerator  Denominator=RPM_to_DC.Denominator
  wires:
  Transfer Fcn1/1 -> Rate Transition/1  "testTF"
  Gain4/1 -> PWM4/1
  Step/1 -> Switch/3
  Rate Transition/1 -> Switch/1  "cont. duty"
  motor arm flag/1 -> Switch/2
  In1/1 -> Transfer Fcn1/1
  Switch/1 -> Gain4/1  "duty"

== system lqr_pos_control/Controller/Control System/RPM_to_DC/Subsystem3 ==
  In1 : Inport
  motor arm flag : Inport  Port=2
  Gain4 : Gain  Gain=2.55
  PWM4 : arduinolib/PWM  pinNumber=5  frequencyType=Specify  desiredFrequency=490.2  achievableFrequency=490.2
  Rate Transition : RateTransition
  Step : Step  Time=.5  Before=99  SampleTime=1/Fs
  Switch : Switch  Threshold=1
  Transfer Fcn1 : TransferFcn  Numerator=RPM_to_DC.Numerator  Denominator=RPM_to_DC.Denominator
  wires:
  Switch/1 -> Gain4/1  "duty"
  In1/1 -> Transfer Fcn1/1
  motor arm flag/1 -> Switch/2
  Rate Transition/1 -> Switch/1  "cont. duty"
  Step/1 -> Switch/3
  Gain4/1 -> PWM4/1
  Transfer Fcn1/1 -> Rate Transition/1  "testTF"

== system lqr_pos_control/Controller/Control System/Flight Controller/State Estimation/Orientation Estimation ==
  IMU : Inport
  realStates : Inport  Port=2
  Demux2 : Demux  Outputs=2
  Kalman : Subsystem  Commented=on
  Madgwick's Complemntary Filter : Subsystem  Commented=on
  Scope : Scope  Commented=on
  Standard Complementary FIlter : Subsystem
  calPoly Kalman : Subsystem  Commented=on
  quaternion Estimate : Outport
  eulerAngleEst : Outport  Port=2
  wires:
  IMU/1 -> Demux2/1
  Madgwick's Complemntary Filter/1(quaternion Estimate) -> quaternion Estimate/1
  Demux2/1 -> Kalman/2(y), calPoly Kalman/1(accel), Madgwick's Complemntary Filter/1(a), Standard Complementary FIlter/1(accIMU)  "a"
  Demux2/2 -> Kalman/1(u), calPoly Kalman/2(gyro), Madgwick's Complemntary Filter/2(w), Standard Complementary FIlter/2(wIMU)  "w"
  Standard Complementary FIlter/1(Orientation Est) -> eulerAngleEst/1  "Comp"
  calPoly Kalman/1(eulerAngle Est) -> Scope/1
  realStates/1 -> ?

== system lqr_pos_control/Controller/Control System/Flight Controller/State Estimation/Subsystem ==
  In1 : Inport
  Enable : EnablePort
  Bus Selector : BusSelector  OutputSignals=Pose.Pose.Position.Z,Pose.Pose.Position.X,Pose.Pose.Position.Y,Twist.Twist.Linear.X,Twist.Twist.Linear.Y,Twist.Twist.Linear.Z
  <Z> : Outport
  <XPos> : Outport  Port=2
  <YPos> : Outport  Port=3
  <Xvel>1 : Outport  Port=4
  <YVel> : Outport  Port=5
  zvel : Outport  Port=6
  wires:
  Bus Selector/3 -> <YPos>/1  "<Y>"
  Bus Selector/1 -> <Z>/1  "<Z>"
  Bus Selector/2 -> <XPos>/1  "<X>"
  Bus Selector/4 -> <Xvel>1/1  "<X>"
  In1/1 -> Bus Selector/1
  Bus Selector/5 -> <YVel>/1  "<Y>"
  Bus Selector/6 -> zvel/1  "<Z>"

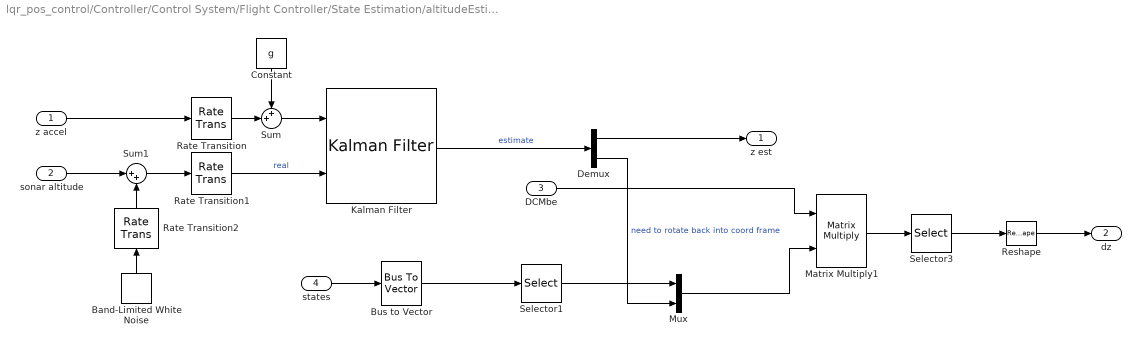
== system lqr_pos_control/Controller/Control System/Flight Controller/State Estimation/altitudeEstimate ==
  z accel : Inport
  sonar altitude : Inport  Port=2
  DCMbe : Inport  Port=3
  states : Inport  Port=4
  Band-Limited White Noise : simulink/Sources/Band-Limited White Noise  Cov=1e-5  Ts=0.1  seed=[23341]
  Bus to Vector : BusToVector
  Constant : Constant  Value=g
  Demux : Demux  Outputs=2
  Kalman Filter : ctrlSharedLib/Kalman Filter  TimeDomain=Discrete-Time  UseCurrentEstimator=on  ModelSource=Individual A, B, C, D matrices  ModelSourceVariable=ss(0.95,1,1,0,1)  A=[1 Ts; 0 1]  B=[Ts*Ts/2;Ts]  C=[1 0]  D=[0]  NumberOfStates=1  NumberOfInputs=1  NumberOfOutputs=1  InitialEstimateSource=Dialog  X0=[0 0]  P0=10  UseK=off  UseGH=on  NumberOfProcessNoiseInputs=1  G=[0 ;1]  TimeInvariantG=on  H=0  TimeInvariantH=on  Q=1  TimeInvariantQ=on  R=.2  TimeInvariantR=on  N=0  TimeInvariantN=on  AddInputPort=on  AddEnablePort=off  OutputEstimatedY=off  OutputP=off  Ts=Ts
  Matrix Multiply1 : Product  Multiplication=Matrix(*)
  Mux : Mux  Inputs=2
  Rate Transition : RateTransition
  Rate Transition1 : RateTransition
  Rate Transition2 : RateTransition
  Reshape : Reshape
  Selector1 : Selector  InputPortWidth=12  IndexOptions=Index vector (dialog)  Indices=[10 12]  OutputSizes=1
  Selector3 : Selector  InputPortWidth=3  IndexOptions=Index vector (dialog)  Indices=3  OutputSizes=1
  Sum : Sum  Inputs=++|
  Sum1 : Sum  Inputs=|++
  z est : Outport
  dz : Outport  Port=2
  wires:
  Demux/1 -> z est/1
  z accel/1 -> Rate Transition/1
  Kalman Filter/1 -> Demux/1  "estimate"
  Rate Transition1/1 -> Kalman Filter/2  "real"
  Rate Transition/1 -> Sum/2
  Constant/1 -> Sum/1
  states/1 -> Bus to Vector/1
  Demux/2 -> Mux/2  "need to rotate back into coord frame"
  Matrix Multiply1/1 -> Selector3/1
  Mux/1 -> Matrix Multiply1/2
  Sum1/1 -> Rate Transition1/1
  DCMbe/1 -> Matrix Multiply1/1
  Sum/1 -> Kalman Filter/1
  Selector3/1 -> Reshape/1
  Bus to Vector/1 -> Selector1/1
  Selector1/1 -> Mux/1
  Reshape/1 -> dz/1
  sonar altitude/1 -> Sum1/1
  Band-Limited White Noise/1 -> Rate Transition2/1
  Rate Transition2/1 -> Sum1/2

== system lqr_pos_control/Controller/Control System/Motor Mixer/Variant Subsystem/Plus Configuration ==
  Constant2 : Constant  Value=airframe.larm
  Constant3 : Constant  Value=airframe.Propeller.Ct
  Constant4 : Constant  Value=airframe.Propeller.Ctau
  MATLAB Function : MATLAB Function  TreatAsAtomicUnit=on
  motorMixing : Outport
  wires:
  Constant2/1 -> MATLAB Function/1(lArm)
  MATLAB Function/1(controlMatInv) -> motorMixing/1
  Constant4/1 -> MATLAB Function/3(CdProp)
  Constant3/1 -> MATLAB Function/2(Ct)

== system lqr_pos_control/Controller/Control System/Motor Mixer/Variant Subsystem/Plus Configuration2 ==
  Constant2 : Constant  Value=airframe.larm
  Constant3 : Constant  Value=airframe.Propeller.Ct
  Constant4 : Constant  Value=airframe.Propeller.Ctau
  MATLAB Function : MATLAB Function  TreatAsAtomicUnit=on
  motorMixing : Outport
  wires:
  Constant3/1 -> MATLAB Function/2(Ct)
  Constant4/1 -> MATLAB Function/3(CdProp)
  MATLAB Function/1(controlMatInv) -> motorMixing/1
  Constant2/1 -> MATLAB Function/1(lArm)

== system lqr_pos_control/Controller/Control System/Motor Mixer/Variant Subsystem/X Configuration ==
  Constant2 : Constant  Value=airframe.larm
  Constant3 : Constant  Value=airframe.Propeller.Ct
  Constant4 : Constant  Value=airframe.Propeller.CdProp
  MATLAB Function : MATLAB Function  TreatAsAtomicUnit=on
  motorMixing : Outport
  wires:
  MATLAB Function/1(controlMatInv) -> motorMixing/1
  Constant3/1 -> MATLAB Function/2(Ct)
  Constant2/1 -> MATLAB Function/1(lArm)
  Constant4/1 -> MATLAB Function/3(CdProp)

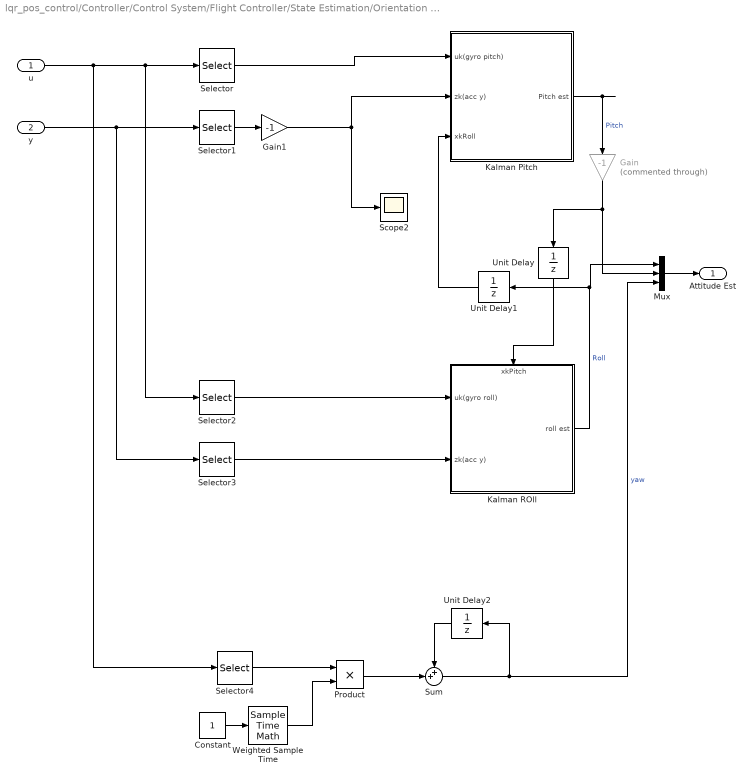
== system lqr_pos_control/Controller/Control System/Flight Controller/State Estimation/Orientation Estimation/Kalman ==
  u : Inport
  y : Inport  Port=2
  Constant : Constant
  Gain : Gain  Commented=through  Gain=-1
  Gain1 : Gain  Gain=-1
  Kalman Pitch : Subsystem
  Kalman ROll : Subsystem
      settings: PortSchema="{\"entries\":[{\"content\":{\"sides\":[{\"content\":{\"connectorIds\":[\"In1\",\"In2\"]},\"type\":\"ConnectorPlacement.EquallySpacedRectSide\",\"uuid\":\"866f8eac-9c5c-472f-897f-b7de637f52da\"},{\"content\":{\"connectorIds\":[\"Out1\"],\"side\":\"RIGHT\"},\"type\":\"ConnectorPlacement.EquallySpacedRectSide\",\"uuid\":\"ce3bd2eb-0be5-45eb-ab3a-703abeb90144\"},{\"content\":{\"connectorIds\":[\"In3\"],\"side\":\"TOP\"},\"type\":\"ConnectorPlacement.EquallySpacedRectSide\",\"uuid\":\"0117a73c-71d3-4471-9333-43b3e528f52d\"}]},\"type\":\"ConnectorPlacement.EquallySpacedConnector\",\"uuid\":\"5e63dce7-8299-4f94-a8bf-df5adfe9ec7c\"}],\"packageUris\":[\"http://schema.mathworks.com/mf0/Connector/R2020b\"],\"version\":\"1.0\"}"
  Mux : Mux  Inputs=3
  Product : Product
  Scope2 : Scope
  Selector : Selector  InputPortWidth=3  IndexOptions=Index vector (dialog)  Indices=[2,3]  OutputSizes=1
  Selector1 : Selector  InputPortWidth=3  IndexOptions=Index vector (dialog)  Indices=1  OutputSizes=1
  Selector2 : Selector  InputPortWidth=3  IndexOptions=Index vector (dialog)  Indices=[1 3]  OutputSizes=1
  Selector3 : Selector  InputPortWidth=3  IndexOptions=Index vector (dialog)  Indices=2  OutputSizes=1
  Selector4 : Selector  InputPortWidth=3  IndexOptions=Index vector (dialog)  Indices=3  OutputSizes=1
  Sum : Sum  Inputs=++|
  Unit Delay : UnitDelay  SampleTime=-1  HasFrameUpgradeWarning=on
  Unit Delay1 : UnitDelay  SampleTime=-1  HasFrameUpgradeWarning=on
  Unit Delay2 : UnitDelay  SampleTime=-1  HasFrameUpgradeWarning=on
  Weighted Sample Time : SampleTimeMath  TsampMathOp=Ts Only
  Attitude Est : Outport
  wires:
  Kalman Pitch/1(Pitch est) -> Gain/1  "Pitch"
  Selector3/1 -> Kalman ROll/2(zk(acc y))
  y/1 -> Selector3/1, Selector1/1
  Kalman ROll/1(roll est) -> Mux/1, Unit Delay1/1  "Roll"
  Selector2/1 -> Kalman ROll/1(uk(gyro roll))
  u/1 -> Selector4/1, Selector2/1, Selector/1
  Mux/1 -> Attitude Est/1
  Constant/1 -> Weighted Sample Time/1
  Weighted Sample Time/1 -> Product/2
  Product/1 -> Sum/2
  Unit Delay2/1 -> Sum/1
  Sum/1 -> Unit Delay2/1, Mux/3  "yaw"
  Selector/1 -> Kalman Pitch/1(uk(gyro pitch))
  Gain/1 -> Unit Delay/1, Mux/2
  Selector4/1 -> Product/1
  Unit Delay/1 -> Kalman ROll/3(xkPitch)
  Unit Delay1/1 -> Kalman Pitch/3(xkRoll)
  Selector1/1 -> Gain1/1
  Gain1/1 -> Scope2/1, Kalman Pitch/2(zk(acc y))

== system lqr_pos_control/Controller/Control System/Flight Controller/State Estimation/Orientation Estimation/Madgwick's Complemntary Filter ==
  note: https://www.x-io.co.uk/res/doc/madgwick_internal_report.pdf
  a : Inport
  w : Inport  Port=2
  Constant : Constant
  Delay One Step2 : Delay  DelayLength=1  InitialCondition=[1 0 0 0]
  Demux3 : Demux
  Gain : Gain
  Gain1 : Gain
  Gain2 : Gain  Gain=-1
  MATLAB Function : MATLAB Function  TreatAsAtomicUnit=on
  Mux1 : Mux
  Quaternions to Rotation Angles : sharedtransform/Quaternions to Rotation Angles  rotationOrder=YXZ  aMode=aMode
      settings: SourceProductBaseCode=AE,PW,DR,MT,UV,VE
  Weighted Sample Time : SampleTimeMath  TsampMathOp=Ts Only
  quaternion Estimate : Outport
  wires:
  Demux3/2 -> Gain/1
  Gain1/1 -> Mux1/3
  Mux1/1 -> Quaternions to Rotation Angles/1, quaternion Estimate/1
  MATLAB Function/1(qEst) -> Delay One Step2/1, Demux3/1
  Gain/1 -> Mux1/2
  Constant/1 -> Weighted Sample Time/1
  Gain2/1 -> Mux1/4
  Weighted Sample Time/1 -> MATLAB Function/3(dt)
  Delay One Step2/1 -> MATLAB Function/4(qIn)
  Demux3/1 -> Mux1/1
  a/1 -> MATLAB Function/1(a)
  Demux3/4 -> Gain2/1
  Demux3/3 -> Gain1/1
  w/1 -> MATLAB Function/2(wB)

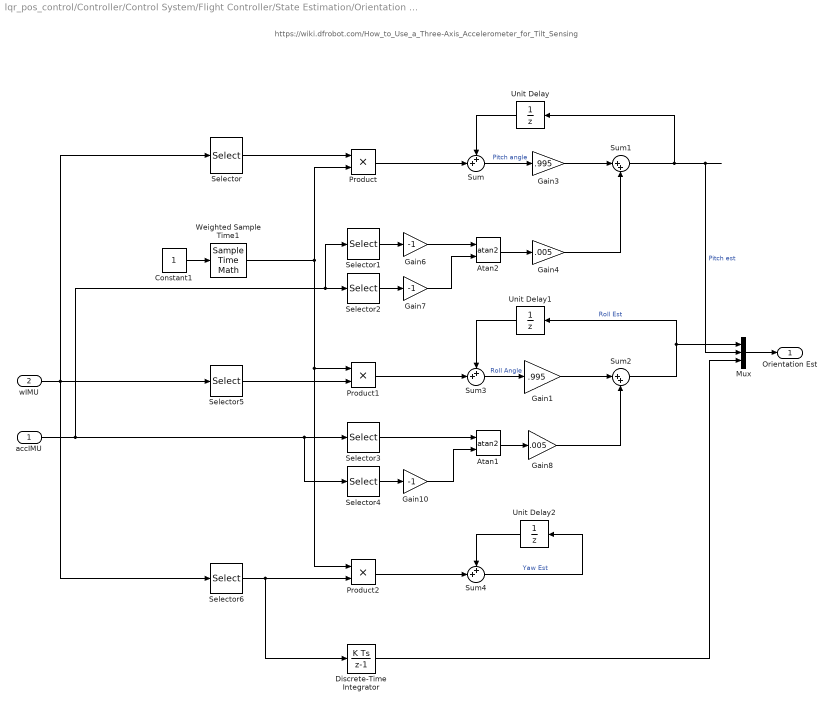
== system lqr_pos_control/Controller/Control System/Flight Controller/State Estimation/Orientation Estimation/Standard Complementary FIlter ==
  note: https://wiki.dfrobot.com/How_to_Use_a_Three-Axis_Accelerometer_for_Tilt_Sensing
  accIMU : Inport
  wIMU : Inport  Port=2
  Atan1 : Trigonometry  Operator=atan2
  Atan2 : Trigonometry  Operator=atan2
  Constant1 : Constant
  Discrete-Time Integrator : DiscreteIntegrator  SampleTime=-1  ICPrevOutput=DiscIntNeverNeededParam  ICPrevScaledInput=DiscIntNeverNeededParam
  Gain1 : Gain  Gain=.995
  Gain10 : Gain  Gain=-1
  Gain3 : Gain  Gain=.995
  Gain4 : Gain  Gain=.005
  Gain6 : Gain  Gain=-1
  Gain7 : Gain  Gain=-1
  Gain8 : Gain  Gain=.005
  Mux : Mux  Inputs=3
  Product : Product
  Product1 : Product
  Product2 : Product
  Selector : Selector  InputPortWidth=3  IndexOptions=Index vector (dialog)  Indices=2  OutputSizes=1
  Selector1 : Selector  InputPortWidth=3  IndexOptions=Index vector (dialog)  Indices=1  OutputSizes=1
  Selector2 : Selector  InputPortWidth=3  IndexOptions=Index vector (dialog)  Indices=3  OutputSizes=1
  Selector3 : Selector  InputPortWidth=3  IndexOptions=Index vector (dialog)  Indices=2  OutputSizes=1
  Selector4 : Selector  InputPortWidth=3  IndexOptions=Index vector (dialog)  Indices=3  OutputSizes=1
  Selector5 : Selector  InputPortWidth=3  IndexOptions=Index vector (dialog)  Indices=1  OutputSizes=1
  Selector6 : Selector  InputPortWidth=3  IndexOptions=Index vector (dialog)  Indices=3  OutputSizes=1
  Sum : Sum  Inputs=++|
  Sum1 : Sum  Inputs=|++
  Sum2 : Sum  Inputs=|++
  Sum3 : Sum  Inputs=++|
  Sum4 : Sum  Inputs=++|
  Unit Delay : UnitDelay  SampleTime=-1  HasFrameUpgradeWarning=on
  Unit Delay1 : UnitDelay  SampleTime=-1  HasFrameUpgradeWarning=on
  Unit Delay2 : UnitDelay  SampleTime=-1  HasFrameUpgradeWarning=on
  Weighted Sample Time1 : SampleTimeMath  TsampMathOp=Ts Only
  Orientation Est : Outport
  wires:
  Gain3/1 -> Sum1/1
  Selector1/1 -> Gain6/1
  accIMU/1 -> Selector3/1, Selector4/1, Selector1/1, Selector2/1
  Selector2/1 -> Gain7/1
  Product/1 -> Sum/2
  Sum1/1 -> Unit Delay/1, Mux/2  "Pitch est"
  Gain7/1 -> Atan2/2
  wIMU/1 -> Selector6/1, Selector5/1, Selector/1
  Atan2/1 -> Gain4/1
  Unit Delay/1 -> Sum/1
  Selector4/1 -> Gain10/1
  Gain10/1 -> Atan1/2
  Atan1/1 -> Gain8/1
  Selector3/1 -> Atan1/1
  Gain4/1 -> Sum1/2
  Constant1/1 -> Weighted Sample Time1/1
  Gain6/1 -> Atan2/1
  Sum/1 -> Gain3/1  "Pitch angle"
  Gain8/1 -> Sum2/2
  Weighted Sample Time1/1 -> Product2/1, Product1/1, Product/2
  Product1/1 -> Sum3/2
  Unit Delay1/1 -> Sum3/1
  Sum3/1 -> Gain1/1  "Roll Angle"
  Gain1/1 -> Sum2/1
  Sum2/1 -> Unit Delay1/1, Mux/1  "Roll Est"
  Unit Delay2/1 -> Sum4/1
  Selector6/1 -> Discrete-Time Integrator/1, Product2/2
  Product2/1 -> Sum4/2
  Sum4/1 -> Unit Delay2/1  "Yaw Est"
  Selector5/1 -> Product1/2
  Mux/1 -> Orientation Est/1
  Selector/1 -> Product/1
  Discrete-Time Integrator/1 -> Mux/3

== system lqr_pos_control/Controller/Control System/Flight Controller/State Estimation/Orientation Estimation/calPoly Kalman ==
  note: https://digitalcommons.calpoly.edu/cgi/viewcontent.cgi?referer=&httpsredir=1&article=1114&context=aerosp
  accel : Inport
  gyro : Inport  Port=2
  Constant : Constant
  Constant1 : Constant  Value=Qkalman
  Constant2 : Constant  Value=Rkalman
  MATLAB Function : MATLAB Function  TreatAsAtomicUnit=on
  Memory1 : Memory  InitialCondition=[Gyro_pitch,Gyro_roll,0]  InheritSampleTime=on
  Memory2 : Memory  InitialCondition=P00  InheritSampleTime=on
  Memory3 : Memory  InitialCondition=P01  InheritSampleTime=on
  Memory4 : Memory  InitialCondition=P11  InheritSampleTime=on
  Scope : Scope
  Weighted Sample Time : SampleTimeMath  TsampMathOp=Ts Only
  eulerAngle Est : Outport
  wires:
  Memory1/1 -> MATLAB Function/3(IC)
  MATLAB Function/2(P00) -> Memory2/1
  Memory2/1 -> MATLAB Function/4("P00 ")
  MATLAB Function/3(P01) -> Memory3/1
  Memory3/1 -> MATLAB Function/5("P01 ")
  MATLAB Function/4(P11) -> Memory4/1
  Memory4/1 -> MATLAB Function/6("P11 ")
  Constant/1 -> Weighted Sample Time/1
  Weighted Sample Time/1 -> MATLAB Function/7(dt)
  Constant1/1 -> MATLAB Function/8(Q)
  Constant2/1 -> MATLAB Function/9(R)
  gyro/1 -> MATLAB Function/2(Gyro_output)
  accel/1 -> MATLAB Function/1(Accel_output)
  MATLAB Function/1(y) -> Memory1/1, eulerAngle Est/1, Scope/1
